simulink model "SIM1"  (R2018b)
settings: Solver=FixedStepAuto  StartTime=0.0  StopTime=10  FixedStep=0.001  RelTol=1e-3  EnableMultiTasking=on
settings Model: Creator=XINGAU  LastModifiedBy=diepn
settings DataIOCC: LimitDataPoints=on
settings OptimizationCC: LifeSpan=inf
settings DebuggingCC: AllowSymbolicDim=off  SFUnexpectedBacktrackingDiag=warning  SFNoUnconditionalDefaultTransitionDiag=warning  SFExecutionAtInitializationDiag=none
settings ModelReferenceCC: PropagateSignalLabelsOutOfModel=off
settings SFSimCC: SimUseLocalCustomCode=off
settings RTWCC: RTWUseLocalCustomCode=off
settings CodeAppCC: StateflowObjectComments=on
settings GRTTargetCC: TargetLangStandard=C89/C90 (ANSI)
settings ConfigComp: CovMetricSettings=dw  CovHtmlReporting=on  CovSaveCumulativeToWorkspaceVar=on  CovSaveSingleToWorkspaceVar=on  CovExternalEMLEnable=off

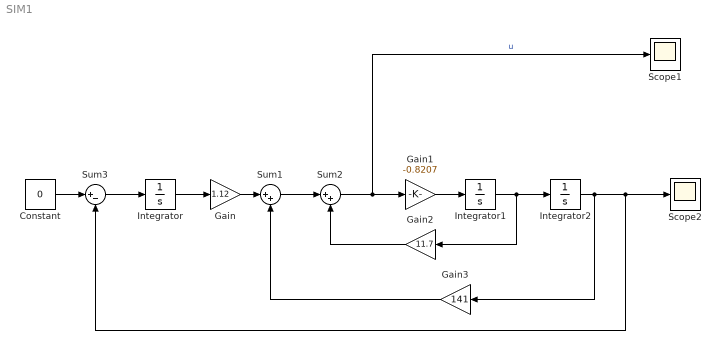
== system SIM1 ==
  Constant : Constant  Value=0
  Gain : Gain  Gain=1.12
  Gain1 : Gain  Gain=-0.8207
  Gain2 : Gain  Gain=11.7
  Gain3 : Gain  Gain=141
  Integrator : Integrator
  Integrator1 : Integrator
  Integrator2 : Integrator  InitialCondition=10
  Scope1 : Scope
  Scope2 : Scope
  Sum1 : Sum  Inputs=|++
  Sum2 : Sum  Inputs=|++
  Sum3 : Sum  Inputs=|+-
  wires:
  Gain/1 -> Sum1/1
  Sum1/1 -> Sum2/1
  Gain1/1 -> Integrator1/1
  Gain2/1 -> Sum2/2
  Gain3/1 -> Sum1/2
  Integrator1/1 -> Gain2/1, Integrator2/1
  Sum2/1 -> Gain1/1, Scope1/1  "u"
  Integrator2/1 -> Sum3/2, Scope2/1, Gain3/1
  Integrator/1 -> Gain/1
  Sum3/1 -> Integrator/1
  Constant/1 -> Sum3/1
